simulink model "isi"  (Simulink 7.0)
settings: Solver=ode45  StartTime=0.0  StopTime=10.0  RelTol=1e-3
libraries: cdsFilt x103, cdsEpicsBinIn x13, cdsEpicsOut x12, cdsMuxMatrix x4, cdsEpicsIn x3, cdsWD x3, cdsRio x2, cdsMatrix x2, dac x1, cdsSwitch x1, cdsParameters x1
(part 1 of 7)
settings Model: Creator=ligo  LastModifiedBy=controls  ExtModeAutoUpdateStatusClock=off
settings DebuggingCC: SaveWithParameterizedLinksMsg=none
settings GRTTargetCC: TargetFcnLib=ansi_tfl_tmw.mat

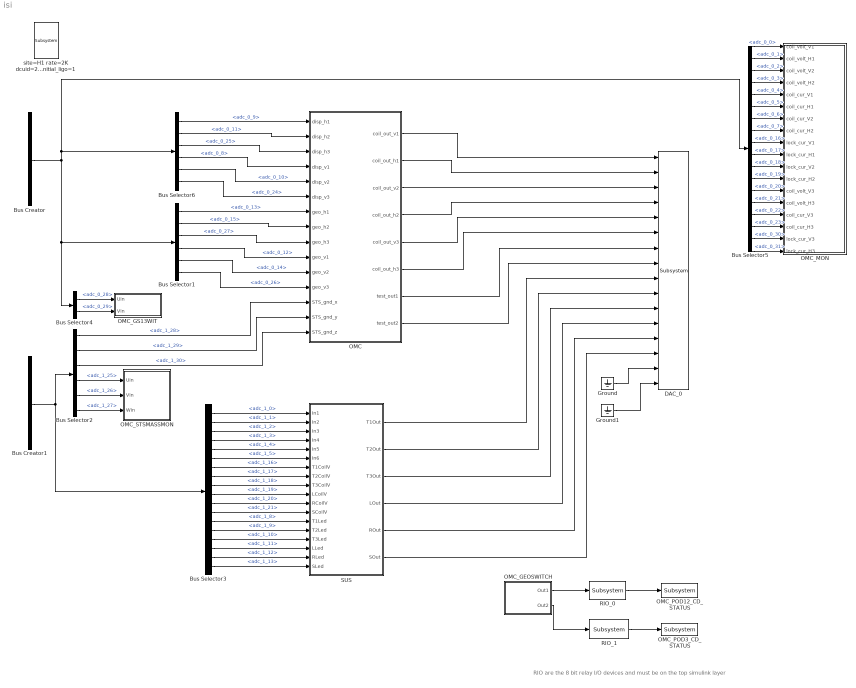
== system isi ==
  note: RIO are the 8 bit relay I/O devices
      | and must be on the top simulink layer
  Bus Creator : BusCreator  Tag=adc_0  Description=ADC0  Inputs='adc_0_0','adc_0_1','adc_0_2','adc_0_3','adc_0_4','adc_0_5','adc_0_6','adc_0_7','adc_0_8','adc_0_9','adc_0_10','adc_0_11','adc_0_12','adc_0_13','adc_0_14','adc_0_15','adc_0_16','adc_0_17','adc_0_18','adc_0_19','adc_0_20','adc_0_21','adc_0_22','adc_0_23','adc_0_24','adc_0_25','adc_0_26','adc_0_27','adc_0_28','adc_0_29','adc_0_30','adc_0_31'
      settings: AttributesFormatString=%<Tag>
  Bus Creator1 : BusCreator  Description=ADC1  Inputs='adc_1_0','adc_1_1','adc_1_2','adc_1_3','adc_1_4','adc_1_5','adc_1_6','adc_1_7','adc_1_8','adc_1_9','adc_1_10','adc_1_11','adc_1_12','adc_1_13','adc_1_14','adc_1_15','adc_1_16','adc_1_17','adc_1_18','adc_1_19','adc_1_20','adc_1_21','adc_1_22','adc_1_23','adc_1_24','adc_1_25','adc_1_26','adc_1_27','adc_1_28','adc_1_29','adc_1_30','adc_1_31'
      settings: AttributesFormatString=%<Description>
  Bus Selector1 : BusSelector  Description=ADC Selector  OutputSignals=adc_0_13,adc_0_15,adc_0_27,adc_0_12,adc_0_14,adc_0_26
      settings: AttributesFormatString=%<Description>
  Bus Selector2 : BusSelector  Description=ADC Selector  OutputSignals=adc_1_28,adc_1_29,adc_1_30,adc_1_25,adc_1_26,adc_1_27
      settings: AttributesFormatString=%<Description>
  Bus Selector3 : BusSelector  Description=ADC Selector  OutputSignals=adc_1_0,adc_1_1,adc_1_2,adc_1_3,adc_1_4,adc_1_5,adc_1_16,adc_1_17,adc_1_18,adc_1_19,adc_1_20,adc_1_21,adc_1_8,adc_1_9,adc_1_10,adc_1_11,adc_1_12,adc_1_13
      settings: AttributesFormatString=%<Description>
  Bus Selector4 : BusSelector  Description=ADC Selector  OutputSignals=adc_0_28,adc_0_29
      settings: AttributesFormatString=%<Description>
  Bus Selector5 : BusSelector  Description=ADC Selector  OutputSignals=adc_0_0,adc_0_1,adc_0_2,adc_0_3,adc_0_4,adc_0_5,adc_0_6,adc_0_7,adc_0_16,adc_0_17,adc_0_18,adc_0_19,adc_0_20,adc_0_21,adc_0_22,adc_0_23,adc_0_30,adc_0_31
      settings: AttributesFormatString=%<Description>
  Bus Selector6 : BusSelector  Description=ADC Selector  OutputSignals=adc_0_9,adc_0_11,adc_0_25,adc_0_8,adc_0_10,adc_0_24
      settings: AttributesFormatString=%<Description>
  DAC_0 : dac/Subsystem  Description=DAC  SystemSampleTime=-1
      settings: AttributesFormatString=%<Description>
  Ground : Ground
  Ground1 : Ground
  OMC : Subsystem
  OMC_GEOSWITCH : Subsystem  Description=GS13 Sensor
      settings: AttributesFormatString=%<Description>
  OMC_GS13WIT : Subsystem
  OMC_MON : Subsystem
  OMC_POD12_CD_STATUS : cdsEpicsOut/Subsystem  Tag=cdsEpicsOutput  Description=|  SystemSampleTime=-1
      | Purpose:                                          
      | Output a FE signal to an EPICS channel.           
      |                                                   
      | Operation:                                        
      | Takes input value and passes it to EPICS record.  
      |                                                   
      | Usage:                                            
      | Name the part with the desired EPICS rrecord name.
      settings: AttributesFormatString=%<Tag>
  OMC_POD3_CD_STATUS : cdsEpicsOut/Subsystem  Tag=cdsEpicsOutput  Description=|  SystemSampleTime=-1
      | Purpose:                                          
      | Output a FE signal to an EPICS channel.           
      |                                                   
      | Operation:                                        
      | Takes input value and passes it to EPICS record.  
      |                                                   
      | Usage:                                            
      | Name the part with the desired EPICS rrecord name.
      settings: AttributesFormatString=%<Tag>
  OMC_STSMASSMON : Subsystem
  RIO_0 : cdsRio/Subsystem  Tag=cdsRio  Description=PCI IIRO 8 relay output and isolated input module  SystemSampleTime=-1
      settings: AttributesFormatString=%<Tag>
  RIO_1 : cdsRio/Subsystem  Tag=cdsRio  Description=PCI IIRO 8 relay output and isolated input module  SystemSampleTime=-1
      settings: AttributesFormatString=%<Tag>
  SUS : Subsystem  Tag=top_names
      settings: AttributesFormatString=%<Tag>
  site=H1 rate=2K dcuid=27 gds_node_id=3 no_sync=1 compat_initial_ligo=1 : cdsParameters/Subsystem  Tag=cdsParameters  SystemSampleTime=-1
      settings: AttributesFormatString=%<Tag>
  wires:
  Bus Creator/1 -> Bus Selector1/1, Bus Selector4/1, Bus Selector6/1, Bus Selector5/1
  OMC_GEOSWITCH/1(Out1) -> RIO_0/1
  OMC_GEOSWITCH/2(Out2) -> RIO_1/1
  RIO_0/1 -> OMC_POD12_CD_STATUS/1
  RIO_1/1 -> OMC_POD3_CD_STATUS/1
  Bus Creator1/1 -> Bus Selector2/1, Bus Selector3/1
  Bus Selector2/4 -> OMC_STSMASSMON/1(Uin)  "<adc_1_25>"
  Bus Selector2/5 -> OMC_STSMASSMON/2(Vin)  "<adc_1_26>"
  Bus Selector2/6 -> OMC_STSMASSMON/3(Win)  "<adc_1_27>"
  Bus Selector3/1 -> SUS/1(In1)  "<adc_1_0>"
  Bus Selector3/2 -> SUS/2(In2)  "<adc_1_1>"
  Bus Selector3/3 -> SUS/3(In3)  "<adc_1_2>"
  Bus Selector3/4 -> SUS/4(In4)  "<adc_1_3>"
  Bus Selector3/5 -> SUS/5(In5)  "<adc_1_4>"
  Bus Selector3/6 -> SUS/6(In6)  "<adc_1_5>"
  Bus Selector3/7 -> SUS/7(T1CoilV)  "<adc_1_16>"
  Bus Selector3/8 -> SUS/8(T2CoilV)  "<adc_1_17>"
  Bus Selector3/9 -> SUS/9(T3CoilV)  "<adc_1_18>"
  Bus Selector3/10 -> SUS/10(LCoilV)  "<adc_1_19>"
  Bus Selector3/11 -> SUS/11(RCoilV)  "<adc_1_20>"
  Bus Selector3/12 -> SUS/12(SCoilV)  "<adc_1_21>"
  Bus Selector3/13 -> SUS/13(T1Led)  "<adc_1_8>"
  Bus Selector3/14 -> SUS/14(T2Led)  "<adc_1_9>"
  Bus Selector3/15 -> SUS/15(T3Led)  "<adc_1_10>"
  Bus Selector3/16 -> SUS/16(LLed)  "<adc_1_11>"
  Bus Selector3/17 -> SUS/17(RLed)  "<adc_1_12>"
  Bus Selector3/18 -> SUS/18(SLed)  "<adc_1_13>"
  Bus Selector2/1 -> OMC/13(STS_gnd_x)  "<adc_1_28>"
  Bus Selector2/2 -> OMC/14(STS_gnd_y)  "<adc_1_29>"
  Bus Selector2/3 -> OMC/15(STS_gnd_z)  "<adc_1_30>"
  OMC/2(coil_out_h1) -> DAC_0/2
  OMC/1(coil_out_v1) -> DAC_0/1
  OMC/4(coil_out_h2) -> DAC_0/4
  OMC/3(coil_out_v2) -> DAC_0/3
  OMC/5(coil_out_v3) -> DAC_0/5
  OMC/8(test_out2) -> DAC_0/8
  SUS/1(T1Out) -> DAC_0/9
  SUS/2(T2Out) -> DAC_0/10
  SUS/3(T3Out) -> DAC_0/11
  SUS/4(LOut) -> DAC_0/12
  SUS/5(ROut) -> DAC_0/13
  SUS/6(SOut) -> DAC_0/14
  Ground/1 -> DAC_0/15
  Ground1/1 -> DAC_0/16
  Bus Selector6/1 -> OMC/1(disp_h1)  "<adc_0_9>"
  Bus Selector6/2 -> OMC/2(disp_h2)  "<adc_0_11>"
  Bus Selector6/3 -> OMC/3(disp_h3)  "<adc_0_25>"
  Bus Selector6/4 -> OMC/4(disp_v1)  "<adc_0_8>"
  Bus Selector6/5 -> OMC/5(disp_v2)  "<adc_0_10>"
  Bus Selector6/6 -> OMC/6(disp_v3)  "<adc_0_24>"
  Bus Selector1/1 -> OMC/7(geo_h1)  "<adc_0_13>"
  Bus Selector1/2 -> OMC/8(geo_h2)  "<adc_0_15>"
  Bus Selector1/3 -> OMC/9(geo_h3)  "<adc_0_27>"
  Bus Selector1/4 -> OMC/10(geo_v1)  "<adc_0_12>"
  Bus Selector1/5 -> OMC/11(geo_v2)  "<adc_0_14>"
  Bus Selector1/6 -> OMC/12(geo_v3)  "<adc_0_26>"
  Bus Selector4/1 -> OMC_GS13WIT/1(Uin)  "<adc_0_28>"
  Bus Selector4/2 -> OMC_GS13WIT/2(Vin)  "<adc_0_29>"
  OMC/6(coil_out_h3) -> DAC_0/6
  OMC/7(test_out1) -> DAC_0/7
  Bus Selector5/1 -> OMC_MON/1(coil_volt_V1)  "<adc_0_0>"
  Bus Selector5/2 -> OMC_MON/2(coil_volt_H1)  "<adc_0_1>"
  Bus Selector5/3 -> OMC_MON/3(coil_volt_V2)  "<adc_0_2>"
  Bus Selector5/4 -> OMC_MON/4(coil_volt_H2)  "<adc_0_3>"
  Bus Selector5/5 -> OMC_MON/5(coil_cur_V1)  "<adc_0_4>"
  Bus Selector5/6 -> OMC_MON/6(coil_cur_H1)  "<adc_0_5>"
  Bus Selector5/7 -> OMC_MON/7(coil_cur_V2)  "<adc_0_6>"
  Bus Selector5/8 -> OMC_MON/8(coil_cur_H2)  "<adc_0_7>"
  Bus Selector5/9 -> OMC_MON/9(lock_cur_V1)  "<adc_0_16>"
  Bus Selector5/10 -> OMC_MON/10(lock_cur_H1)  "<adc_0_17>"
  Bus Selector5/11 -> OMC_MON/11(lock_cur_V2)  "<adc_0_18>"
  Bus Selector5/12 -> OMC_MON/12(lock_cur_H2)  "<adc_0_19>"
  Bus Selector5/13 -> OMC_MON/13(coil_volt_V3)  "<adc_0_20>"
  Bus Selector5/14 -> OMC_MON/14(coil_volt_H3)  "<adc_0_21>"
  Bus Selector5/15 -> OMC_MON/15(coil_cur_V3)  "<adc_0_22>"
  Bus Selector5/16 -> OMC_MON/16(coil_cur_H3)  "<adc_0_23>"
  Bus Selector5/17 -> OMC_MON/17(lock_cur_V3)  "<adc_0_30>"
  Bus Selector5/18 -> OMC_MON/18(lock_cur_H3)  "<adc_0_31>"

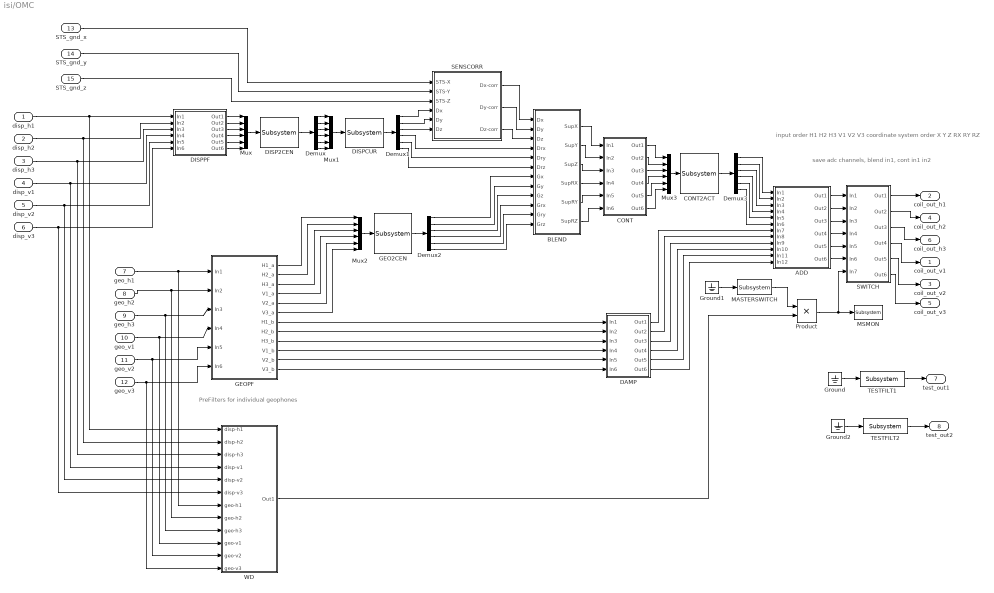
== system isi/OMC ==
  note: input order
      | H1 H2 H3 V1 V2 V3
      |
      | coordinate system order
      | X Y Z RX RY RZ
  note: save adc channels, blend in1, cont in1 in2
  note: PreFilters for
      | individual geophones
  disp_h1 : Inport  OutDataType=sfix(16)  OutScaling=2^0
  disp_h2 : Inport  Port=2  OutDataType=sfix(16)  OutScaling=2^0
  disp_h3 : Inport  Port=3  OutDataType=sfix(16)  OutScaling=2^0
  disp_v1 : Inport  Port=4  OutDataType=sfix(16)  OutScaling=2^0
  disp_v2 : Inport  Port=5  OutDataType=sfix(16)  OutScaling=2^0
  disp_v3 : Inport  Port=6  OutDataType=sfix(16)  OutScaling=2^0
  geo_h1 : Inport  Port=7  OutDataType=sfix(16)  OutScaling=2^0
  geo_h2 : Inport  Port=8  OutDataType=sfix(16)  OutScaling=2^0
  geo_h3 : Inport  Port=9  OutDataType=sfix(16)  OutScaling=2^0
  geo_v1 : Inport  Port=10  OutDataType=sfix(16)  OutScaling=2^0
  geo_v2 : Inport  Port=11  OutDataType=sfix(16)  OutScaling=2^0
  geo_v3 : Inport  Port=12  OutDataType=sfix(16)  OutScaling=2^0
  STS_gnd_x : Inport  Port=13  OutDataType=sfix(16)  OutScaling=2^0
  STS_gnd_y : Inport  Port=14  OutDataType=sfix(16)  OutScaling=2^0
  STS_gnd_z : Inport  Port=15  OutDataType=sfix(16)  OutScaling=2^0
  ADD : Subsystem
  BLEND : Subsystem
  CONT : Subsystem
  CONT2ACT : cdsMuxMatrix/Subsystem  Tag=cdsMuxMatrix  Description=Any size matrix. Inputs and outputs must be connected using Mux and Demux parts.  SystemSampleTime=-1
      settings: AttributesFormatString=%<Tag>
  DAMP : Subsystem
  DISP2CEN : cdsMuxMatrix/Subsystem  Tag=cdsMuxMatrix  Description=Any size matrix. Inputs and outputs must be connected using Mux and Demux parts.  SystemSampleTime=-1
      settings: AttributesFormatString=%<Tag>
  DISPCUR : cdsMuxMatrix/Subsystem  Tag=cdsMuxMatrix  Description=Any size matrix. Inputs and outputs must be connected using Mux and Demux parts.  SystemSampleTime=-1
      settings: AttributesFormatString=%<Tag>
  DISPPF : Subsystem
  Demux{,1..3} (4 alike) : Demux  Outputs=6
  GEO2CEN : cdsMuxMatrix/Subsystem  Tag=cdsMuxMatrix  Description=Any size matrix. Inputs and outputs must be connected using Mux and Demux parts.  SystemSampleTime=-1
      settings: AttributesFormatString=%<Tag>
  GEOPF : Subsystem
  Ground : Ground
  Ground1 : Ground
  Ground2 : Ground
  MASTERSWITCH : cdsEpicsBinIn/Subsystem  Tag=cdsEpicsBinIn  Description=|  SystemSampleTime=-1
      | Purpose:                                                                            
      | Create an EPICS binary (0 or 1) input channel to the FE realtime controls.          
      |                                                                                     
      | Operation:                                                                          
      | Outputs value from an EPICS ai record. Value is binary input (bi Epics record type).
      |                                                                                     
      | Usage:                                                                              
      | Name the part with the desired EPICS channel name.
      settings: AttributesFormatString=%<Tag>
  MSMON : cdsEpicsOut/Subsystem  Tag=cdsEpicsOutput  Description=|  SystemSampleTime=-1
      | Purpose:                                          
      | Output a FE signal to an EPICS channel.           
      |                                                   
      | Operation:                                        
      | Takes input value and passes it to EPICS record.  
      |                                                   
      | Usage:                                            
      | Name the part with the desired EPICS rrecord name.
      settings: AttributesFormatString=%<Tag>
  Mux{,1..3} (4 alike) : Mux  Inputs=6
  Product : Product  OutDataType=sfix(16)  OutScaling=2^0  RndMeth=Zero
  SENSCORR : Subsystem
  SWITCH : Subsystem
  TESTFILT1 : cdsFilt/Subsystem  Tag=cdsFilt  Description=|  SystemSampleTime=-1
      | Purpose:                                                                                                                                                                                                                                  
      | Standard CDS IIR filter module.                                                                                                                                                                                                           
      |                                                                                                                                                                                                                                           
      | Operation:                                                                                                                                                                                                                                
      | Consists of 10 second order section IIR filters, plus a ramped gain stage. In FE code, also provides pre-defined test points and excitation channel inputs. The filter coefficients are defined in the LIGO system using the 'foton' tool.
      |                                                                                                                                                                                                                                           
      | Usage:                                                                                                                                                                                                                                    
      | Name the part with the desired filter module name.
      settings: AttributesFormatString=%<Tag>
  TESTFILT2 : cdsFilt/Subsystem  Tag=cdsFilt  Description=|  SystemSampleTime=-1
      | Purpose:                                                                                                                                                                                                                                  
      | Standard CDS IIR filter module.                                                                                                                                                                                                           
      |                                                                                                                                                                                                                                           
      | Operation:                                                                                                                                                                                                                                
      | Consists of 10 second order section IIR filters, plus a ramped gain stage. In FE code, also provides pre-defined test points and excitation channel inputs. The filter coefficients are defined in the LIGO system using the 'foton' tool.
      |                                                                                                                                                                                                                                           
      | Usage:                                                                                                                                                                                                                                    
      | Name the part with the desired filter module name.
      settings: AttributesFormatString=%<Tag>
  WD : Subsystem
  coil_out_v1 : Outport  OutDataType=sfix(16)  OutScaling=2^0
  coil_out_h1 : Outport  Port=2  OutDataType=sfix(16)  OutScaling=2^0
  coil_out_v2 : Outport  Port=3  OutDataType=sfix(16)  OutScaling=2^0
  coil_out_h2 : Outport  Port=4  OutDataType=sfix(16)  OutScaling=2^0
  coil_out_v3 : Outport  Port=5  OutDataType=sfix(16)  OutScaling=2^0
  coil_out_h3 : Outport  Port=6  OutDataType=sfix(16)  OutScaling=2^0
  test_out1 : Outport  Port=7  OutDataType=sfix(16)  OutScaling=2^0
  test_out2 : Outport  Port=8  OutDataType=sfix(16)  OutScaling=2^0
  wires:
  Mux/1 -> DISP2CEN/1
  DISP2CEN/1 -> Demux/1
  DISPCUR/1 -> Demux1/1
  Mux2/1 -> GEO2CEN/1
  GEO2CEN/1 -> Demux2/1
  Mux3/1 -> CONT2ACT/1
  CONT2ACT/1 -> Demux3/1
  DISPPF/1(Out1) -> Mux/1
  DISPPF/2(Out2) -> Mux/2
  DISPPF/3(Out3) -> Mux/3
  DISPPF/4(Out4) -> Mux/4
  DISPPF/5(Out5) -> Mux/5
  DISPPF/6(Out6) -> Mux/6
  DAMP/1(Out1) -> ADD/7(In7)
  DAMP/2(Out2) -> ADD/8(In8)
  DAMP/3(Out3) -> ADD/9(In9)
  DAMP/4(Out4) -> ADD/10(In10)
  DAMP/5(Out5) -> ADD/11(In11)
  DAMP/6(Out6) -> ADD/12(In12)
  Demux3/1 -> ADD/1(In1)
  Demux3/2 -> ADD/2(In2)
  Demux3/3 -> ADD/3(In3)
  Demux3/4 -> ADD/4(In4)
  Demux3/5 -> ADD/5(In5)
  Demux3/6 -> ADD/6(In6)
  ADD/1(Out1) -> SWITCH/1(In1)
  ADD/2(Out2) -> SWITCH/2(In2)
  ADD/3(Out3) -> SWITCH/3(In3)
  ADD/4(Out4) -> SWITCH/4(In4)
  ADD/5(Out5) -> SWITCH/5(In5)
  ADD/6(Out6) -> SWITCH/6(In6)
  Demux1/4 -> BLEND/4(Drx)
  Demux1/5 -> BLEND/5(Dry)
  Demux1/6 -> BLEND/6(Drz)
  Demux2/1 -> BLEND/7(Gx)
  Demux2/2 -> BLEND/8(Gy)
  Demux2/3 -> BLEND/9(Gz)
  Demux2/4 -> BLEND/10(Grx)
  Demux2/5 -> BLEND/11(Gry)
  Demux2/6 -> BLEND/12(Grz)
  BLEND/1(SupX) -> CONT/1(In1)
  BLEND/2(SupY) -> CONT/2(In2)
  BLEND/3(SupZ) -> CONT/3(In3)
  BLEND/4(SupRX) -> CONT/4(In4)
  BLEND/5(SupRY) -> CONT/5(In5)
  BLEND/6(SupRZ) -> CONT/6(In6)
  CONT/1(Out1) -> Mux3/1
  CONT/2(Out2) -> Mux3/2
  CONT/3(Out3) -> Mux3/3
  CONT/4(Out4) -> Mux3/4
  CONT/5(Out5) -> Mux3/5
  CONT/6(Out6) -> Mux3/6
  SWITCH/1(Out1) -> coil_out_h1/1
  SWITCH/2(Out2) -> coil_out_h2/1
  SWITCH/3(Out3) -> coil_out_h3/1
  SWITCH/4(Out4) -> coil_out_v1/1
  SWITCH/5(Out5) -> coil_out_v2/1
  SWITCH/6(Out6) -> coil_out_v3/1
  Ground1/1 -> MASTERSWITCH/1
  disp_h1/1 -> DISPPF/1(In1), WD/1(disp-h1)
  disp_h2/1 -> DISPPF/2(In2), WD/2(disp-h2)
  disp_h3/1 -> DISPPF/3(In3), WD/3(disp-h3)
  disp_v1/1 -> DISPPF/4(In4), WD/4(disp-v1)
  disp_v2/1 -> DISPPF/5(In5), WD/5(disp-v2)
  disp_v3/1 -> DISPPF/6(In6), WD/6(disp-v3)
  geo_h1/1 -> GEOPF/1(In1), WD/7(geo-h1)
  geo_h2/1 -> GEOPF/2(In2), WD/8(geo-h2)
  geo_h3/1 -> GEOPF/3(In3), WD/9(geo-h3)
  geo_v1/1 -> GEOPF/4(In4), WD/10(geo-v1)
  geo_v2/1 -> GEOPF/5(In5), WD/11(geo-v2)
  geo_v3/1 -> GEOPF/6(In6), WD/12(geo-v3)
  GEOPF/1(H1_a) -> Mux2/1
  GEOPF/2(H2_a) -> Mux2/2
  GEOPF/3(H3_a) -> Mux2/3
  GEOPF/4(V1_a) -> Mux2/4
  GEOPF/5(V2_a) -> Mux2/5
  GEOPF/6(V3_a) -> Mux2/6
  GEOPF/7(H1_b) -> DAMP/1(In1)
  GEOPF/8(H2_b) -> DAMP/2(In2)
  GEOPF/9(H3_b) -> DAMP/3(In3)
  GEOPF/10(V1_b) -> DAMP/4(In4)
  GEOPF/11(V2_b) -> DAMP/5(In5)
  GEOPF/12(V3_b) -> DAMP/6(In6)
  Mux1/1 -> DISPCUR/1
  Demux/1 -> Mux1/1
  Demux/2 -> Mux1/2
  Demux/3 -> Mux1/3
  Demux/4 -> Mux1/4
  Demux/5 -> Mux1/5
  Demux/6 -> Mux1/6
  STS_gnd_x/1 -> SENSCORR/1(STS-X)
  STS_gnd_y/1 -> SENSCORR/2(STS-Y)
  STS_gnd_z/1 -> SENSCORR/3(STS-Z)
  Demux1/1 -> SENSCORR/4(Dx)
  Demux1/2 -> SENSCORR/5(Dy)
  Demux1/3 -> SENSCORR/6(Dz)
  SENSCORR/1(Dx-corr) -> BLEND/1(Dx)
  SENSCORR/2(Dy-corr) -> BLEND/2(Dy)
  SENSCORR/3(Dz-corr) -> BLEND/3(Dz)
  MASTERSWITCH/1 -> Product/1
  Product/1 -> SWITCH/7(In7), MSMON/1
  WD/1(Out1) -> Product/2
  Ground/1 -> TESTFILT1/1
  TESTFILT1/1 -> test_out1/1
  Ground2/1 -> TESTFILT2/1
  TESTFILT2/1 -> test_out2/1

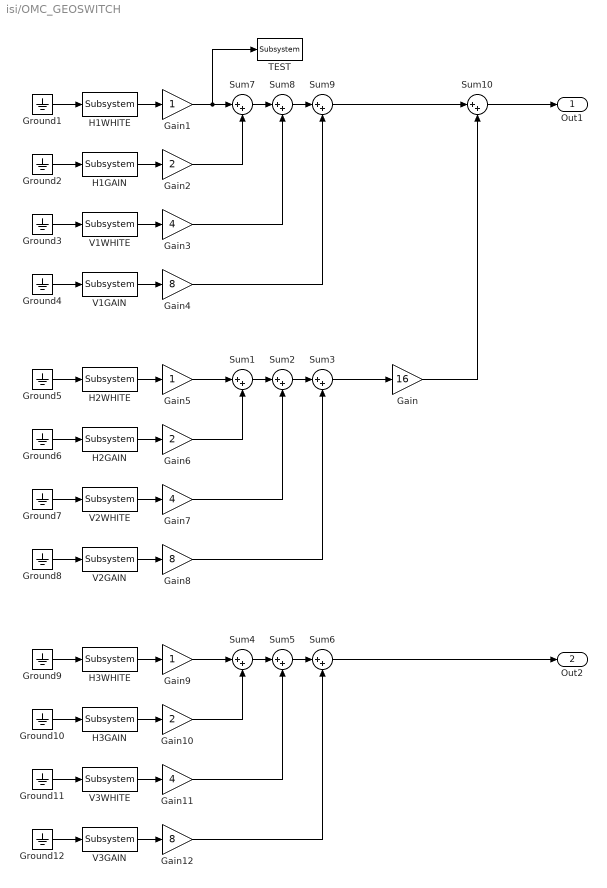
== system isi/OMC_GEOSWITCH ==
  Gain : Gain  Gain=16  ParameterDataType=sfix(16)  ParameterScaling=2^0  OutDataType=sfix(16)  OutScaling=2^0
  Gain1 : Gain  ParameterDataType=sfix(16)  ParameterScaling=2^0  OutDataType=sfix(16)  OutScaling=2^0
  Gain10 : Gain  Gain=2  ParameterDataType=sfix(16)  ParameterScaling=2^0  OutDataType=sfix(16)  OutScaling=2^0
  Gain11 : Gain  Gain=4  ParameterDataType=sfix(16)  ParameterScaling=2^0  OutDataType=sfix(16)  OutScaling=2^0
  Gain12 : Gain  Gain=8  ParameterDataType=sfix(16)  ParameterScaling=2^0  OutDataType=sfix(16)  OutScaling=2^0
  Gain2 : Gain  Gain=2  ParameterDataType=sfix(16)  ParameterScaling=2^0  OutDataType=sfix(16)  OutScaling=2^0
  Gain3 : Gain  Gain=4  ParameterDataType=sfix(16)  ParameterScaling=2^0  OutDataType=sfix(16)  OutScaling=2^0
  Gain4 : Gain  Gain=8  ParameterDataType=sfix(16)  ParameterScaling=2^0  OutDataType=sfix(16)  OutScaling=2^0
  Gain5 : Gain  ParameterDataType=sfix(16)  ParameterScaling=2^0  OutDataType=sfix(16)  OutScaling=2^0
  Gain6 : Gain  Gain=2  ParameterDataType=sfix(16)  ParameterScaling=2^0  OutDataType=sfix(16)  OutScaling=2^0
  Gain7 : Gain  Gain=4  ParameterDataType=sfix(16)  ParameterScaling=2^0  OutDataType=sfix(16)  OutScaling=2^0
  Gain8 : Gain  Gain=8  ParameterDataType=sfix(16)  ParameterScaling=2^0  OutDataType=sfix(16)  OutScaling=2^0
  Gain9 : Gain  ParameterDataType=sfix(16)  ParameterScaling=2^0  OutDataType=sfix(16)  OutScaling=2^0
  Ground{1..12} (12 alike) : Ground
  H1GAIN : cdsEpicsBinIn/Subsystem  Tag=cdsEpicsBinIn  Description=|  SystemSampleTime=-1
      | Purpose:                                                                            
      | Create an EPICS binary (0 or 1) input channel to the FE realtime controls.          
      |                                                                                     
      | Operation:                                                                          
      | Outputs value from an EPICS ai record. Value is binary input (bi Epics record type).
      |                                                                                     
      | Usage:                                                                              
      | Name the part with the desired EPICS channel name.
      settings: AttributesFormatString=%<Tag>
  H1WHITE : cdsEpicsBinIn/Subsystem  Tag=cdsEpicsBinIn  Description=|  SystemSampleTime=-1
      | Purpose:                                                                            
      | Create an EPICS binary (0 or 1) input channel to the FE realtime controls.          
      |                                                                                     
      | Operation:                                                                          
      | Outputs value from an EPICS ai record. Value is binary input (bi Epics record type).
      |                                                                                     
      | Usage:                                                                              
      | Name the part with the desired EPICS channel name.
      settings: AttributesFormatString=%<Tag>
  H2GAIN : cdsEpicsBinIn/Subsystem  Tag=cdsEpicsBinIn  Description=|  SystemSampleTime=-1
      | Purpose:                                                                            
      | Create an EPICS binary (0 or 1) input channel to the FE realtime controls.          
      |                                                                                     
      | Operation:                                                                          
      | Outputs value from an EPICS ai record. Value is binary input (bi Epics record type).
      |                                                                                     
      | Usage:                                                                              
      | Name the part with the desired EPICS channel name.
      settings: AttributesFormatString=%<Tag>
  H2WHITE : cdsEpicsBinIn/Subsystem  Tag=cdsEpicsBinIn  Description=|  SystemSampleTime=-1
      | Purpose:                                                                            
      | Create an EPICS binary (0 or 1) input channel to the FE realtime controls.          
      |                                                                                     
      | Operation:                                                                          
      | Outputs value from an EPICS ai record. Value is binary input (bi Epics record type).
      |                                                                                     
      | Usage:                                                                              
      | Name the part with the desired EPICS channel name.
      settings: AttributesFormatString=%<Tag>
  H3GAIN : cdsEpicsBinIn/Subsystem  Tag=cdsEpicsBinIn  Description=|  SystemSampleTime=-1
      | Purpose:                                                                            
      | Create an EPICS binary (0 or 1) input channel to the FE realtime controls.          
      |                                                                                     
      | Operation:                                                                          
      | Outputs value from an EPICS ai record. Value is binary input (bi Epics record type).
      |                                                                                     
      | Usage:                                                                              
      | Name the part with the desired EPICS channel name.
      settings: AttributesFormatString=%<Tag>
  H3WHITE : cdsEpicsBinIn/Subsystem  Tag=cdsEpicsBinIn  Description=|  SystemSampleTime=-1
      | Purpose:                                                                            
      | Create an EPICS binary (0 or 1) input channel to the FE realtime controls.          
      |                                                                                     
      | Operation:                                                                          
      | Outputs value from an EPICS ai record. Value is binary input (bi Epics record type).
      |                                                                                     
      | Usage:                                                                              
      | Name the part with the desired EPICS channel name.
      settings: AttributesFormatString=%<Tag>
  Sum{1..10} (10 alike) : Sum  Inputs=|++  OutDataType=sfix(16)  OutScaling=2^0
  TEST : cdsEpicsOut/Subsystem  Tag=cdsEpicsOutput  Description=|  SystemSampleTime=-1
      | Purpose:                                          
      | Output a FE signal to an EPICS channel.           
      |                                                   
      | Operation:                                        
      | Takes input value and passes it to EPICS record.  
      |                                                   
      | Usage:                                            
      | Name the part with the desired EPICS rrecord name.
      settings: AttributesFormatString=%<Tag>
  V1GAIN : cdsEpicsBinIn/Subsystem  Tag=cdsEpicsBinIn  Description=|  SystemSampleTime=-1
      | Purpose:                                                                            
      | Create an EPICS binary (0 or 1) input channel to the FE realtime controls.          
      |                                                                                     
      | Operation:                                                                          
      | Outputs value from an EPICS ai record. Value is binary input (bi Epics record type).
      |                                                                                     
      | Usage:                                                                              
      | Name the part with the desired EPICS channel name.
      settings: AttributesFormatString=%<Tag>
  V1WHITE : cdsEpicsBinIn/Subsystem  Tag=cdsEpicsBinIn  Description=|  SystemSampleTime=-1
      | Purpose:                                                                            
      | Create an EPICS binary (0 or 1) input channel to the FE realtime controls.          
      |                                                                                     
      | Operation:                                                                          
      | Outputs value from an EPICS ai record. Value is binary input (bi Epics record type).
      |                                                                                     
      | Usage:                                                                              
      | Name the part with the desired EPICS channel name.
      settings: AttributesFormatString=%<Tag>
  V2GAIN : cdsEpicsBinIn/Subsystem  Tag=cdsEpicsBinIn  Description=|  SystemSampleTime=-1
      | Purpose:                                                                            
      | Create an EPICS binary (0 or 1) input channel to the FE realtime controls.          
      |                                                                                     
      | Operation:                                                                          
      | Outputs value from an EPICS ai record. Value is binary input (bi Epics record type).
      |                                                                                     
      | Usage:                                                                              
      | Name the part with the desired EPICS channel name.
      settings: AttributesFormatString=%<Tag>
  V2WHITE : cdsEpicsBinIn/Subsystem  Tag=cdsEpicsBinIn  Description=|  SystemSampleTime=-1
      | Purpose:                                                                            
      | Create an EPICS binary (0 or 1) input channel to the FE realtime controls.          
      |                                                                                     
      | Operation:                                                                          
      | Outputs value from an EPICS ai record. Value is binary input (bi Epics record type).
      |                                                                                     
      | Usage:                                                                              
      | Name the part with the desired EPICS channel name.
      settings: AttributesFormatString=%<Tag>
  V3GAIN : cdsEpicsBinIn/Subsystem  Tag=cdsEpicsBinIn  Description=|  SystemSampleTime=-1
      | Purpose:                                                                            
      | Create an EPICS binary (0 or 1) input channel to the FE realtime controls.          
      |                                                                                     
      | Operation:                                                                          
      | Outputs value from an EPICS ai record. Value is binary input (bi Epics record type).
      |                                                                                     
      | Usage:                                                                              
      | Name the part with the desired EPICS channel name.
      settings: AttributesFormatString=%<Tag>
  V3WHITE : cdsEpicsBinIn/Subsystem  Tag=cdsEpicsBinIn  Description=|  SystemSampleTime=-1
      | Purpose:                                                                            
      | Create an EPICS binary (0 or 1) input channel to the FE realtime controls.          
      |                                                                                     
      | Operation:                                                                          
      | Outputs value from an EPICS ai record. Value is binary input (bi Epics record type).
      |                                                                                     
      | Usage:                                                                              
      | Name the part with the desired EPICS channel name.
      settings: AttributesFormatString=%<Tag>
  Out1 : Outport  OutDataType=sfix(16)  OutScaling=2^0
  Out2 : Outport  Port=2  OutDataType=sfix(16)  OutScaling=2^0
  wires:
  Gain/1 -> Sum10/2
  Sum10/1 -> Out1/1
  Sum9/1 -> Sum10/1
  Ground10/1 -> H3GAIN/1
  Ground11/1 -> V3WHITE/1
  Ground12/1 -> V3GAIN/1
  Ground9/1 -> H3WHITE/1
  Gain12/1 -> Sum6/2
  Sum6/1 -> Out2/1
  Sum5/1 -> Sum6/1
  V3GAIN/1 -> Gain12/1
  Gain11/1 -> Sum5/2
  Sum4/1 -> Sum5/1
  V3WHITE/1 -> Gain11/1
  H3WHITE/1 -> Gain9/1
  Gain9/1 -> Sum4/1
  H3GAIN/1 -> Gain10/1
  Gain10/1 -> Sum4/2
  Ground6/1 -> H2GAIN/1
  Ground7/1 -> V2WHITE/1
  Ground8/1 -> V2GAIN/1
  Ground5/1 -> H2WHITE/1
  Gain8/1 -> Sum3/2
  Sum3/1 -> Gain/1
  Sum2/1 -> Sum3/1
  V2GAIN/1 -> Gain8/1
  Gain7/1 -> Sum2/2
  Sum1/1 -> Sum2/1
  V2WHITE/1 -> Gain7/1
  H2WHITE/1 -> Gain5/1
  Gain5/1 -> Sum1/1
  H2GAIN/1 -> Gain6/1
  Gain6/1 -> Sum1/2
  Ground2/1 -> H1GAIN/1
  Ground3/1 -> V1WHITE/1
  Ground4/1 -> V1GAIN/1
  Ground1/1 -> H1WHITE/1
  Gain4/1 -> Sum9/2
  Sum8/1 -> Sum9/1
  V1GAIN/1 -> Gain4/1
  Gain3/1 -> Sum8/2
  Sum7/1 -> Sum8/1
  V1WHITE/1 -> Gain3/1
  H1WHITE/1 -> Gain1/1
  Gain1/1 -> TEST/1, Sum7/1
  H1GAIN/1 -> Gain2/1
  Gain2/1 -> Sum7/2

== system isi/OMC_GS13WIT ==
  Uin : Inport  OutDataType=sfix(16)  OutScaling=2^0
  Vin : Inport  Port=2  OutDataType=sfix(16)  OutScaling=2^0
  A : cdsFilt/Subsystem  Tag=cdsFilt  Description=|  SystemSampleTime=-1
      | Purpose:                                                                                                                                                                                                                                  
      | Standard CDS IIR filter module.                                                                                                                                                                                                           
      |                                                                                                                                                                                                                                           
      | Operation:                                                                                                                                                                                                                                
      | Consists of 10 second order section IIR filters, plus a ramped gain stage. In FE code, also provides pre-defined test points and excitation channel inputs. The filter coefficients are defined in the LIGO system using the 'foton' tool.
      |                                                                                                                                                                                                                                           
      | Usage:                                                                                                                                                                                                                                    
      | Name the part with the desired filter module name.
      settings: AttributesFormatString=%<Tag>
  B : cdsFilt/Subsystem  Tag=cdsFilt  Description=|  SystemSampleTime=-1
      | Purpose:                                                                                                                                                                                                                                  
      | Standard CDS IIR filter module.                                                                                                                                                                                                           
      |                                                                                                                                                                                                                                           
      | Operation:                                                                                                                                                                                                                                
      | Consists of 10 second order section IIR filters, plus a ramped gain stage. In FE code, also provides pre-defined test points and excitation channel inputs. The filter coefficients are defined in the LIGO system using the 'foton' tool.
      |                                                                                                                                                                                                                                           
      | Usage:                                                                                                                                                                                                                                    
      | Name the part with the desired filter module name.
      settings: AttributesFormatString=%<Tag>
  Terminator3 : Terminator
  Terminator4 : Terminator
  wires:
  Uin/1 -> A/1
  A/1 -> Terminator3/1
  Vin/1 -> B/1
  B/1 -> Terminator4/1
